simulink model "sfcndemo_sfun_fcncall"  (Simulink 7.6)
settings: Solver=FixedStepDiscrete  SolverMode=SingleTasking  StartTime=0.0  StopTime=1  FixedStep=.1  RelTol=1e-3  AbsTol=1e-6
Description:
  | Function-call generator C-MEX S-function
settings Model: Creator=The MathWorks Inc.  ExtModeTrigMode=oneshot  ExtModeArmWhenConnect=off  ExtModeAutoUpdateStatusClock=off
settings DataIOCC: LimitDataPoints=off  SignalLoggingName=sigsOut
settings OptimizationCC: BooleanDataType=off  InlineInvariantSignals=on  InitFltsAndDblsToZero=on
settings DebuggingCC: SaveWithParameterizedLinksMsg=none  SignalResolutionControl=TryResolveAllWithWarning  SolverPrmCheckMsg=none  InheritedTsInSrcMsg=none  MultiTaskDSMMsg=warning  MultiTaskCondExecSysMsg=none
settings HardwareCC: TargetUnknown=on
settings RTWCC: IncludeERTFirstTime=on
settings CodeAppCC: CustomSymbolStrFcn=$F$N$M
settings GRTTargetCC: TargetFcnLib=ansi_tfl_tmw.mat

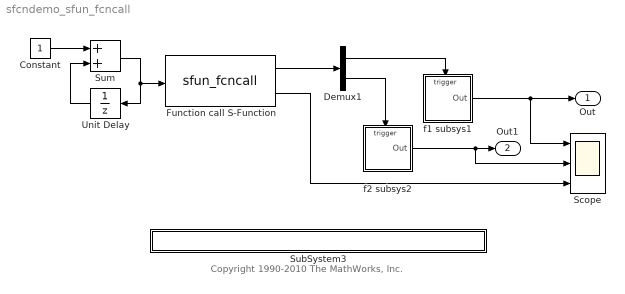
== system sfcndemo_sfun_fcncall ==
  note: Copyright 1990-2010 The MathWorks, Inc.
  Constant : Constant
  Demux1 : Demux  Outputs=2
  Function call S-Function : S-Function  FunctionName=sfun_fcncall  EnableBusSupport=off
      mask Type: S-function: sfun_fcncall
      mask Description: This is a S-function block which is configured to execute "function-call" subsystems on the 1st and 2nd elements of the 1st output port. Note that function-calls can be issued from the 1st output port only.
  Scope : Scope  NumInputPorts=3
      settings: TimeRange=1  YMin=0~0~0  YMax=1~10~10
  SubSystem3 : Subsystem  mask{filename=sfun_fcncall.c}
      mask init:
      | x=sfundemo_maskdisp;
      settings: AttributesFormatString=\n  OpenFcn=sfundemo_openfcn
      mask Display: disp(x);
  Sum : Sum  SaturateOnIntegerOverflow=on  InputSameDT=on  OutDataTypeStr=Inherit: Same as first input
  Unit Delay : UnitDelay  SampleTime=.1
  f1 subsys1 : Subsystem  TreatAsAtomicUnit=on
  f2 subsys2 : Subsystem  TreatAsAtomicUnit=on
  Out : Outport  InitialOutput=0
  Out1 : Outport  Port=2  InitialOutput=0
  wires:
  Sum/1 -> Unit Delay/1, Function call S-Function/1
  Demux1/2 -> f2 subsys2/Trigger
  Function call S-Function/1 -> Demux1/1
  Constant/1 -> Sum/1
  Unit Delay/1 -> Sum/2
  f1 subsys1/1(Out) -> Out/1, Scope/1
  Demux1/1 -> f1 subsys1/Trigger
  Function call S-Function/2 -> Scope/3
  f2 subsys2/1(Out) -> Out1/1, Scope/2

== system sfcndemo_sfun_fcncall/SubSystem3 ==

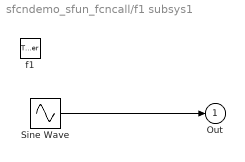
== system sfcndemo_sfun_fcncall/f1 subsys1 ==
  f1 : TriggerPort  TriggerType=function-call
  Sine Wave : Sin
  Out : Outport  InitialOutput=0
  wires:
  Sine Wave/1 -> Out/1

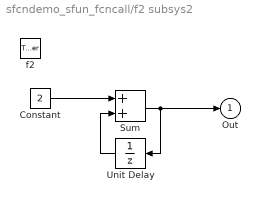
== system sfcndemo_sfun_fcncall/f2 subsys2 ==
  f2 : TriggerPort  TriggerType=function-call
  Constant : Constant  Value=2
  Sum : Sum  SaturateOnIntegerOverflow=on  InputSameDT=on  OutDataTypeStr=Inherit: Same as first input
  Unit Delay : UnitDelay  SampleTime=-1
  Out : Outport  InitialOutput=0
  wires:
  Constant/1 -> Sum/1
  Unit Delay/1 -> Sum/2
  Sum/1 -> Unit Delay/1, Out/1
